simulink model "CellModel"  (R2022a)
settings: Solver=ode3  StartTime=0.0  StopTime=sim_duration  FixedStep=simulation.setup.stepsize  RelTol=1e-3  EnableMultiTasking=on
values from neighbouring files (symbols this model uses):
  Q = cellCapacity * 3600    [Model_3RC.m]
undefined symbols (not defined in the file or in its folder): initStates, parameters
settings Model: PauseTimes=4328.31  PacingRate=1000  Creator=Wenlin  LastModifiedBy=Wenlin
settings DebuggingCC: UnconnectedInputMsg=warning  UnconnectedOutputMsg=warning  UnconnectedLineMsg=warning
settings RTWCC: DLArmComputeVersion=19.05

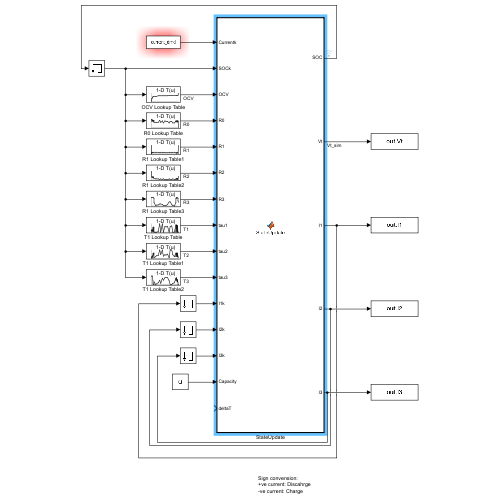
[thumbnail: Simulink's stored preview of the top-level diagram]
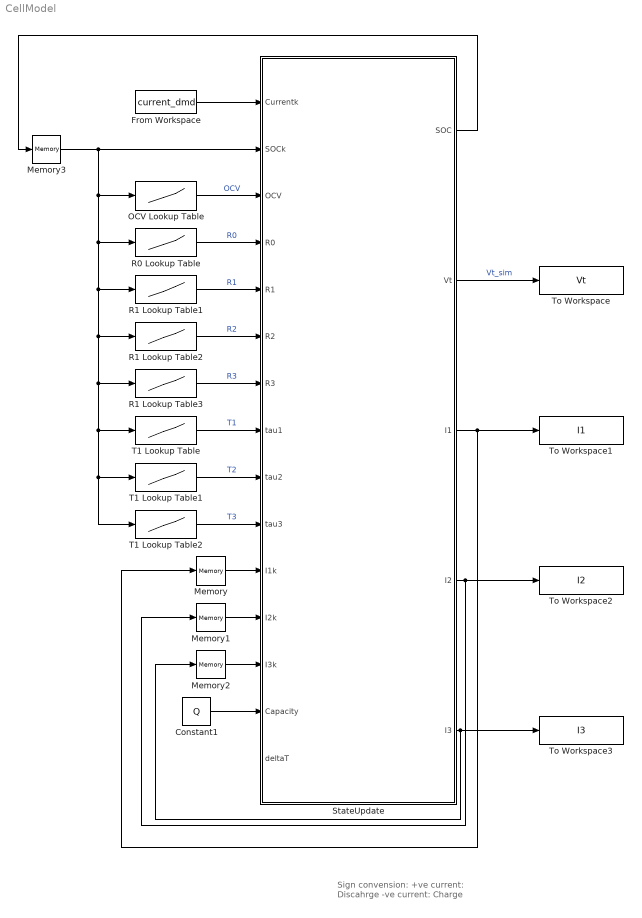
== system CellModel ==
  note: Sign convension:
      | +ve current: Discahrge
      | -ve current: Charge
  Constant1 : Constant  Value=Q
  From Workspace : FromWorkspace  VariableName=current_dmd
  Memory : Memory  InitialCondition=initStates.I_RC(1)
  Memory1 : Memory  InitialCondition=initStates.I_RC(2)
  Memory2 : Memory  InitialCondition=initStates.I_RC(3)
  Memory3 : Memory  InitialCondition=initStates.SOC
  OCV Lookup Table : Lookup_n-D  NumberOfTableDimensions=1  BreakpointsForDimension1=parameters.SOC  Table=parameters.OCV  ExtrapMethod=Clip  UseLastTableValue=on  InternalRulePriority=Speed  RndMeth=Simplest
  R0 Lookup Table : Lookup_n-D  NumberOfTableDimensions=1  BreakpointsForDimension1=parameters.SOC  Table=parameters.R0  ExtrapMethod=Clip  UseLastTableValue=on  InternalRulePriority=Speed  RndMeth=Simplest
  R1 Lookup Table1 : Lookup_n-D  NumberOfTableDimensions=1  BreakpointsForDimension1=parameters.SOC  Table=parameters.R1  ExtrapMethod=Clip  UseLastTableValue=on  InternalRulePriority=Speed  RndMeth=Simplest
  R1 Lookup Table2 : Lookup_n-D  NumberOfTableDimensions=1  BreakpointsForDimension1=parameters.SOC  Table=parameters.R2  ExtrapMethod=Clip  UseLastTableValue=on  InternalRulePriority=Speed  RndMeth=Simplest
  R1 Lookup Table3 : Lookup_n-D  NumberOfTableDimensions=1  BreakpointsForDimension1=parameters.SOC  Table=parameters.R3  ExtrapMethod=Clip  UseLastTableValue=on  InternalRulePriority=Speed  RndMeth=Simplest
  StateUpdate : MATLAB Function  TreatAsAtomicUnit=on
  T1 Lookup Table : Lookup_n-D  NumberOfTableDimensions=1  BreakpointsForDimension1=parameters.SOC  Table=parameters.T1  ExtrapMethod=Clip  UseLastTableValue=on  InternalRulePriority=Speed  RndMeth=Simplest
  T1 Lookup Table1 : Lookup_n-D  NumberOfTableDimensions=1  BreakpointsForDimension1=parameters.SOC  Table=parameters.T2  ExtrapMethod=Clip  UseLastTableValue=on  InternalRulePriority=Speed  RndMeth=Simplest
  T1 Lookup Table2 : Lookup_n-D  NumberOfTableDimensions=1  BreakpointsForDimension1=parameters.SOC  Table=parameters.T3  ExtrapMethod=Clip  UseLastTableValue=on  InternalRulePriority=Speed  RndMeth=Simplest
  To Workspace : ToWorkspace  VariableName=Vt  SaveFormat=Timeseries  SampleTime=-1
  To Workspace1 : ToWorkspace  VariableName=I1  SaveFormat=Timeseries  SampleTime=-1
  To Workspace2 : ToWorkspace  VariableName=I2  SaveFormat=Timeseries  SampleTime=-1
  To Workspace3 : ToWorkspace  VariableName=I3  SaveFormat=Timeseries  SampleTime=-1
  wires:
  From Workspace/1 -> StateUpdate/1(Currentk)
  StateUpdate/3(I1) -> Memory/1, To Workspace1/1
  Memory1/1 -> StateUpdate/12(I2k)
  StateUpdate/4(I2) -> Memory1/1, To Workspace2/1
  Memory3/1 -> R1 Lookup Table2/1, R1 Lookup Table3/1, T1 Lookup Table2/1, T1 Lookup Table1/1, T1 Lookup Table/1, R1 Lookup Table1/1, R0 Lookup Table/1, OCV Lookup Table/1, StateUpdate/2(SOCk)
  Memory2/1 -> StateUpdate/13(I3k)
  Constant1/1 -> StateUpdate/14(Capacity)
  R1 Lookup Table3/1 -> StateUpdate/7(R3)  "R3"
  T1 Lookup Table1/1 -> StateUpdate/9(tau2)  "T2"
  StateUpdate/5(I3) -> To Workspace3/1, Memory2/1
  Memory/1 -> StateUpdate/11(I1k)
  R0 Lookup Table/1 -> StateUpdate/4(R0)  "R0"
  R1 Lookup Table1/1 -> StateUpdate/5(R1)  "R1"
  R1 Lookup Table2/1 -> StateUpdate/6(R2)  "R2"
  T1 Lookup Table/1 -> StateUpdate/8(tau1)  "T1"
  T1 Lookup Table2/1 -> StateUpdate/10(tau3)  "T3"
  StateUpdate/1(SOC) -> Memory3/1
  OCV Lookup Table/1 -> StateUpdate/3(OCV)  "OCV"
  StateUpdate/2(Vt) -> To Workspace/1  "Vt_sim"

== matlab function CellModel/StateUpdate ==
  data: Currentk input; SOC output; SOCk input; OCV input; R0 input; R1 input; R2 input; R3 input; tau1 input; tau2 input; tau3 input; I1k input; I2k input; I3k input; Capacity input; deltaT input; Vt output; I1 output; I2 output; I3 output
function [SOC, Vt, I1, I2, I3] = StateUpdate(Currentk, SOCk, OCV, R0, R1, R2, R3, tau1, tau2, tau3, I1k, I2k, I3k, Capacity, deltaT)

    Q = Capacity*3600;

    % Calculate currents
    I1 =  ( 1 - exp(-deltaT/tau1) ) * Currentk + exp(-deltaT/tau1) * I1k;
    I2 =  ( 1 - exp(-deltaT/tau2) ) * Currentk + exp(-deltaT/tau2) * I2k;
    I3 =  ( 1 - exp(-deltaT/tau3) ) * Currentk + exp(-deltaT/tau3) * I3k;

    % Update voltage & SOC
    Vt   = OCV - (R0*Currentk) - R1*I1 - R2*I2 - R3*I3;
    SOC  = SOCk - (deltaT/Q) * Currentk;

end
